simulink model "unary_numerical_integration"  (R2016b)
settings: Solver=ode45  StartTime=realmin  StopTime=pi  RelTol=1e-3
settings Model: Creator=frederick_hsu  LastModifiedBy=frederick_hsu

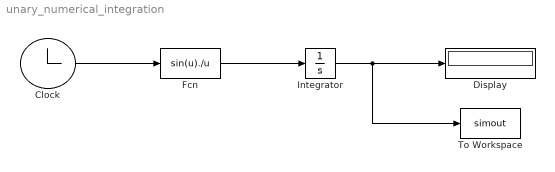
== system unary_numerical_integration ==
  Clock : Clock
      settings: Decimation=3
  Display : Display
      settings: Decimation=5
  Fcn : Fcn  Expr=sin(u)./u
  Integrator : Integrator
  To Workspace : ToWorkspace  VariableName=simout  SaveFormat=Timeseries  SampleTime=-1
  wires:
  Clock/1 -> Fcn/1
  Fcn/1 -> Integrator/1
  Integrator/1 -> To Workspace/1, Display/1
